simulink model "MAGBOJOS_NO. 3"  (R2024a)
settings: Solver=VariableStepAuto  StartTime=0.0  StopTime=20.0  RelTol=1e-3
values from neighbouring files (symbols this model uses):
  G_den = [1 2 3 4 5 6 7 1]    [ILAGAN_NO. 5.m]    (also in ILAGAN_NO. 6.m = [1 2 3 4 1]; MAGBOJOS_NO. 3.m = [1 2 1]; MAGBOJOS_NO. 4.m = [2 1])
  G_num = [8 7 6 5 4 3 2]    [ILAGAN_NO. 5.m]    (also in ILAGAN_NO. 6.m = [4 3 2 1]; MAGBOJOS_NO. 3.m = [1]; MAGBOJOS_NO. 4.m = [1])
settings Model: Creator=Acer  LastModifiedBy=Acer

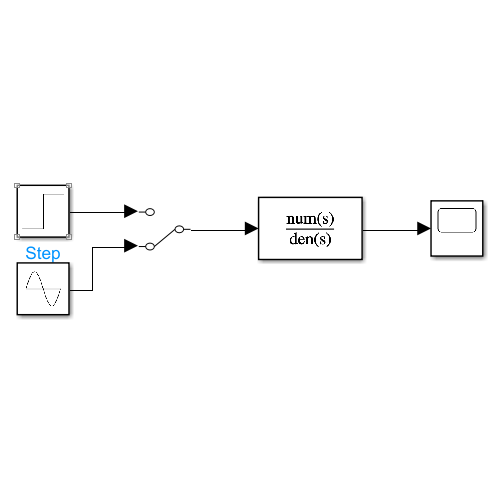
[thumbnail: Simulink's stored preview of the top-level diagram]
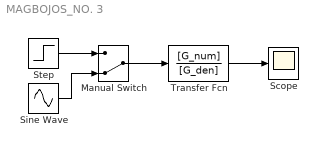
== system MAGBOJOS_NO. 3 ==
  Manual Switch : ManualSwitch  CurrentSetting=0
  Scope : Scope
  Sine Wave : Sin  SampleTime=0
  Step : Step  SampleTime=0
  Transfer Fcn : TransferFcn  Numerator=[G_num]  Denominator=[G_den]
  wires:
  Step/1 -> Manual Switch/1
  Manual Switch/1 -> Transfer Fcn/1
  Sine Wave/1 -> Manual Switch/2
  Transfer Fcn/1 -> Scope/1
